simulink model "encoder"  (R2023b)
settings: Solver=VariableStepAuto  StartTime=0.0  StopTime=10.0  RelTol=1e-3
settings Model: Creator=Acer  LastModifiedBy=sabat
settings SolverCC: AlgebraicLoopSolver=TrustRegion
settings DebuggingCC: UnconnectedInputMsg=warning  UnconnectedOutputMsg=warning  UnconnectedLineMsg=warning
settings ModelReferenceCC: EnableRefExpFcnMdlSchedulingChecks=on

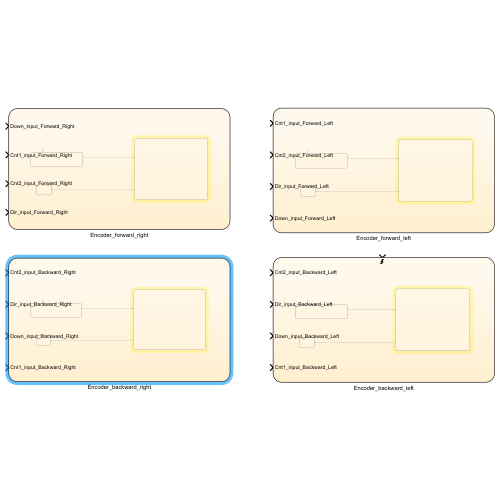
[thumbnail: Simulink's stored preview of the top-level diagram]
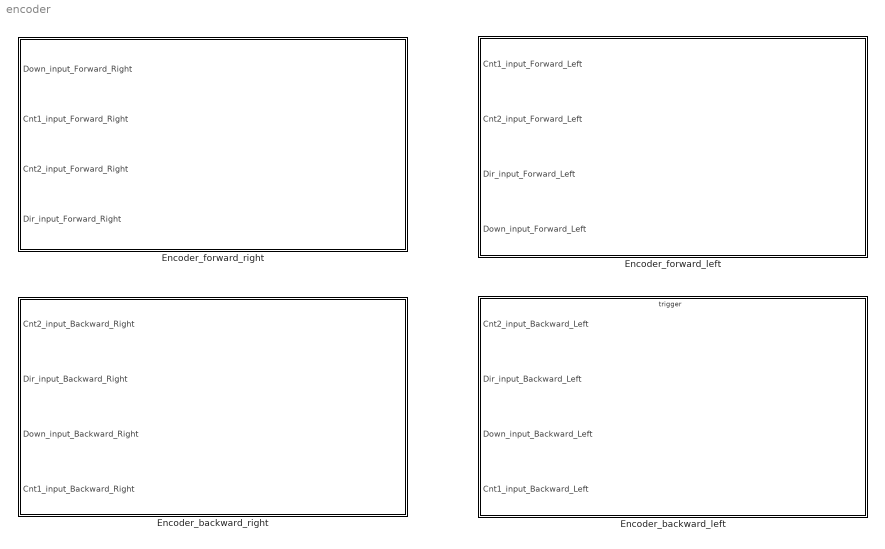
== system encoder ==
  Encoder_backward_left : Stateflow chart  TreatAsAtomicUnit=on
  Encoder_backward_right : Stateflow chart  TreatAsAtomicUnit=on
  Encoder_forward_left : Stateflow chart  TreatAsAtomicUnit=on
  Encoder_forward_right : Stateflow chart  TreatAsAtomicUnit=on

== stateflow chart encoder/Encoder_backward_left ==
  state Read
    cnt2_Backward_Left = Cnt2_input_Backward_Left;
    Dir_Backward_Left = Dir_input_Backward_Left;
    Down_Backward_Left =Down_input_Backward_Left;
    if  Down_Backward_Left
    if (cnt2_Backward_Left < cnt1_Backward_Left)
    diff_Backward_Left = cnt1_Backward_Left - cnt2_Backward_Left;
    else
    diff_Backward_Left = (65535 - cnt2_Backward_Left) + cnt1_Backward_Left;
    end
    else
    if (cnt2_Backward_Left > cnt1_Backward_Left)
    diff _Backward_Right= cnt2_Backward_Right - cnt1_Backward_Right;
    else
    diff _Backward_Right= (65535 - cnt1_Backward_Right) + cnt2_Backward_Right;
    end
    end
    speed _Backward_Right= diff_Backward_Right / PPR / 60
  state Start
    cnt1_Backward_Left = Cnt1_input_Backward_Left
  state End
  (default) -> Start
  Start -> Read : [after(300, msec)]
  Read -> End : {send(Encoder_Backward_Left,Read_Inputs_State.Logic)}
  data: PPR constant double =12; Cnt2_input_Backward_Left input; Dir_input_Backward_Left input; Down_input_Backward_Left input; Dir_Backward_Left local; diff_Backward_Left local; Down_Backward_Left local; cnt1_Backward_Left local; cnt2_Backward_Left local; speed local; Cnt1_input_Backward_Left input
  events: Encoder_Backward_Left input RISING_EDGE_EVENT

== stateflow chart encoder/Encoder_forward_left ==
  state Read
    cnt2_Forward_Left = Cnt2_input_Forward_Left;
    Dir_Forward_Left = Dir_input_Forward_Left;
    Down_Forward_Left =Down_input_Forward_Left;
    if  Down_Forward_Left
    if (cnt2_Forward_Left < cnt1_Forward_Left)
    diff_Forward_Left= cnt1_Forward_Left- cnt2_Forward_Left;
    else
    diff_Forward_Left = (65535 - cnt2_Forward_Left) + cnt1_Forward_Left;
    end
    else
    if (cnt2_Forward_Left > cnt1_Forward_Leftt)
    diff _Forward_Left= cnt2_Forward_Left - cnt1_Forward_Left;
    else
    diff _Forward_Left= (65535 - cnt1_Forward_Left) + cnt2_Forward_Left;
    end
    end
    speed _Forward_Left= diff_Forward_Left / PPR / 60
  state Start
    cnt1_Forward_Left = Cnt1_input_Forward_Left
  state End
  (default) -> Start
  Start -> Read : [after(300, msec)]
  Read -> End : {send(Encoder_Forward_Left,Read_Inputs_State.Logic)}
  data: PPR constant double =12; Cnt1_input_Forward_Left input; Cnt2_input_Forward_Left input; Dir_input_Forward_Left input; Down_input_Forward_Left input; cnt1_Forward_Leftt local; speed local; Dir_Forward_Left local; diff_Forward_Left local; Down_Forward_Left local; cnt1_Forward_Left local; cnt2_Forward_Left local
  events: Encoder_Forward_Left local FUNCTION_CALL_EVENT

== stateflow chart encoder/Encoder_backward_right ==
  state Read
    cnt2_Backward_Right = Cnt2_input_Backward_Right;
    Dir_Backward_Right = Dir_input_Backward_Right;
    Down_Backward_Right =Down_input_Backward_Right;
    if  Down_Backward_Right
    if (cnt2_Backward_Right < cnt1_Backward_Right)
    diff_Backward_Right = cnt1_Backward_Right - cnt2_Backward_Right;
    else
    diff_Backward_Right = (65535 - cnt2_Backward_Right) + cnt1_Backward_Right;
    end
    else
    if (cnt2_Backward_Right > cnt1_Backward_Right)
    diff _Backward_Right= cnt2_Backward_Right - cnt1_Backward_Right;
    else
    diff _Backward_Right= (65535 - cnt1_Backward_Right) + cnt2_Backward_Right;
    end
    end
    speed _Backward_Right= diff_Backward_Right / PPR / 60
  state Start
    cnt1_Backward_Right = Cnt1_input_Backward_Right
  state End
  (default) -> Start
  Start -> Read : [after(300, msec)]
  Read -> End : {send(Encoder_Backward_Right,Read_Inputs_State.Logic)}
  data: PPR constant double =12; Cnt2_input_Backward_Right input; Dir_input_Backward_Right input; Down_input_Backward_Right input; Dir_Backward_Right local; diff_Backward_Right local; Down_Backward_Right local; cnt1_Backward_Right local; cnt2_Backward_Right local; Cnt1_input_Backward_Right input
  events: Encoder_Backward_Right local FUNCTION_CALL_EVENT

== stateflow chart encoder/Encoder_forward_right ==
  state Read
    cnt2_Forward_Right = Cnt2_input_Forward_Right;
    Dir_Forward_Right = Dir_input_Forward_Right;
    Down_Forward_Right =Down_input_Forward_Right;
    if  Down_Forward_Right
    if (cnt2_Forward_Right < cnt1_Forward_Right)
    diff_Forward_Right = cnt1_Forward_Right - cnt2_Forward_Right;
    else
    diff_Forward_Right = (65535 - cnt2_Forward_Right) + cnt1_Forward_Right;
    end
    else
    if (cnt2_Forward_Right > cnt1_Forward_Right)
    diff _Forward_Right= cnt2_Forward_Right - cnt1_Forward_Right;
    else
    diff _Forward_Right= (65535 - cnt1_Forward_Right) + cnt2_Forward_Right;
    end
    end
    speed _Forward_Right= diff_Forward_Right / PPR / 60;
  state Start
    cnt1_Forward_Right = Cnt1_input_Forward_Right
  state End
  (default) -> Start
  Start -> Read : [after(300, msec)]
  Read -> End : {send(Encoder_Forward_Right,Read_Inputs_State.Logic)}
  data: diff_Forward_Right local; Down_Forward_Right local; Down_input_Forward_Right input; cnt1_Forward_Right local; cnt2_Forward_Right local; Cnt1_input_Forward_Right input; Cnt2_input_Forward_Right input; Dir_input_Forward_Right input; Dir_Forward_Right local; speed local; PPR constant double =12; speed_Forward_Right local
  events: Encoder_Forward_Right local FUNCTION_CALL_EVENT
